simulink model "quad_control"  (R2017a)
settings: Solver=ode3  StartTime=0.0  StopTime=100  FixedStep=0.01  RelTol=1e-3  EnableMultiTasking=on
values from neighbouring files (symbols this model uses):
  g = 9.8    [init.m]
  m = 0.445    [init.m]
undefined symbols (not defined in the file or in its folder): allocate, altitude_control, attitude_control, fault_estimate, faults, model, position_control, sliding_var, sliding_var_z
libraries: simulink x2
settings Model: Creator=smishra  LastModifiedBy=Bharath
settings DataIOCC: LimitDataPoints=on  SaveFormat=Array  Refine=5
settings OptimizationCC: LifeSpan=inf
settings DebuggingCC: SFUnexpectedBacktrackingDiag=warning  SFNoUnconditionalDefaultTransitionDiag=warning  SFExecutionAtInitializationDiag=none
settings HardwareCC: ProdBitPerPointer=32  ProdBitPerSizeT=32  ProdBitPerPtrDiffT=32  ProdLargestAtomicFloat=None  ProdIntDivRoundTo=Undefined  ProdEndianess=Unspecified  ProdWordSize=32  ProdHWDeviceType=32-bit Generic
settings ModelReferenceCC: PropagateSignalLabelsOutOfModel=off
settings GRTTargetCC: TargetLangStandard=C89/C90 (ANSI)  GeneratePreprocessorConditionals=Disable all
settings ConfigComp: CovMetricSettings=dw  CovHtmlReporting=on  CovSaveCumulativeToWorkspaceVar=on  CovSaveSingleToWorkspaceVar=on  CovExternalEMLEnable=off

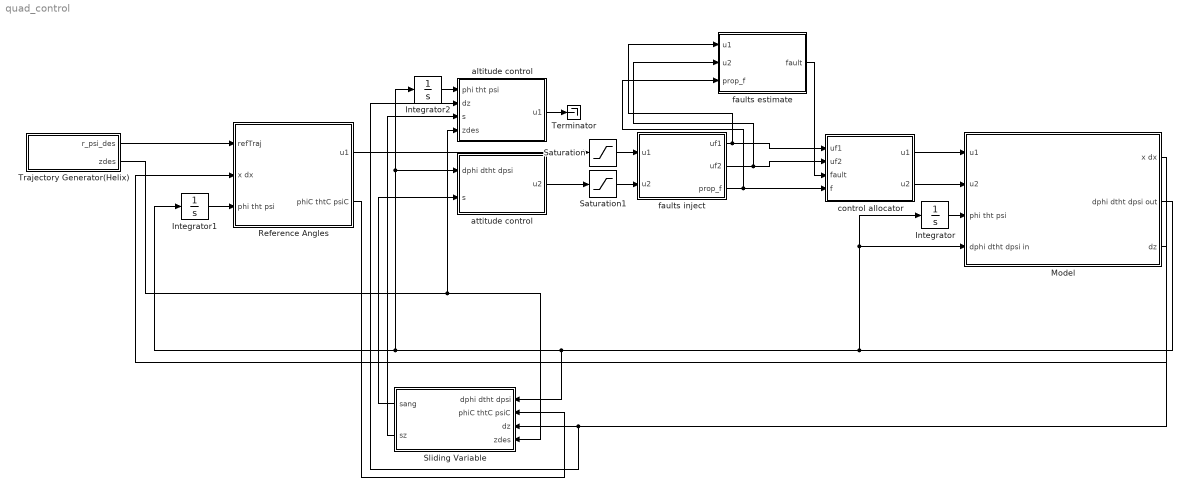
== system quad_control ==
  Integrator : Integrator
  Integrator1 : Integrator
  Integrator2 : Integrator
  Model : Subsystem
  Reference Angles : Subsystem
  Saturation : Saturate  UpperLimit=2*m*g  LowerLimit=0
  Saturation1 : Saturate  UpperLimit=0.2  LowerLimit=-0.2
  Sliding Variable : Subsystem
  Terminator : Terminator
  Trajectory Generator(Helix) : Subsystem
  altitude control : Subsystem
  attitude control : Subsystem
  control allocator : Subsystem
  faults estimate : Subsystem
  faults inject : Subsystem
  wires:
  Trajectory Generator(Helix)/1(r_psi_des) -> Reference Angles/1(refTraj)
  Model/2(dphi dtht dpsi out) -> Model/4(dphi dtht dpsi in), Integrator/1, Sliding Variable/1(dphi dtht dpsi), Integrator1/1, attitude control/1(dphi dtht dpsi), Integrator2/1
  Integrator/1 -> Model/3(phi tht psi)
  Integrator1/1 -> Reference Angles/3(phi tht psi)
  Model/1(x dx) -> Reference Angles/2(x dx)
  Sliding Variable/1(sang) -> attitude control/2(s)
  Reference Angles/2(phiC thtC psiC) -> Sliding Variable/2(phiC thtC psiC)
  Reference Angles/1(u1) -> Saturation/1
  attitude control/1(u2) -> Saturation1/1
  Trajectory Generator(Helix)/2(zdes) -> altitude control/4(zdes), Sliding Variable/4(zdes)
  Model/3(dz) -> altitude control/2(dz), Sliding Variable/3(dz)
  Sliding Variable/2(sz) -> altitude control/3(s)
  altitude control/1(u1) -> Terminator/1
  Integrator2/1 -> altitude control/1(phi tht psi)
  Saturation/1 -> faults inject/1(u1)
  Saturation1/1 -> faults inject/2(u2)
  control allocator/1(u1) -> Model/1(u1)
  control allocator/2(u2) -> Model/2(u2)
  faults estimate/1(fault) -> control allocator/3(fault)
  faults inject/1(uf1) -> faults estimate/1(u1), control allocator/1(uf1)
  faults inject/2(uf2) -> faults estimate/2(u2), control allocator/2(uf2)
  faults inject/3(prop_f) -> control allocator/4(f), faults estimate/3(prop_f)

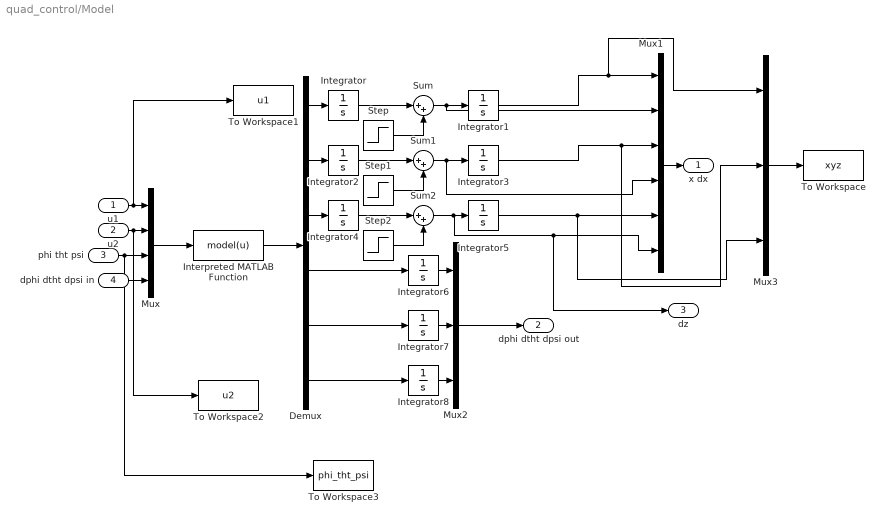
== system quad_control/Model ==
  u1 : Inport
  u2 : Inport  Port=2
  phi tht psi : Inport  Port=3
  dphi dtht dpsi in : Inport  Port=4
  Demux : Demux  Outputs=6
  Integrator{,1..2,4,6..8} (7 alike) : Integrator
  Integrator3 : Integrator  InitialCondition=8
  Integrator5 : Integrator  InitialCondition=8
  Interpreted MATLAB Function : MATLABFcn  MATLABFcn=model(u)  OutputDimensions=6
  Mux : Mux
  Mux1 : Mux  Inputs=6
  Mux2 : Mux  Inputs=3
  Mux3 : Mux  Inputs=3
  Step : Step  Time=025  After=0  SampleTime=0
  Step1 : Step  Time=25  After=0  SampleTime=0
  Step2 : Step  Time=25  After=0  SampleTime=0
  Sum : Sum  Inputs=|++
  Sum1 : Sum  Inputs=|++
  Sum2 : Sum  Inputs=|++
  To Workspace : ToWorkspace  VariableName=xyz  SampleTime=-1
  To Workspace1 : ToWorkspace  VariableName=u1  SampleTime=-1
  To Workspace2 : ToWorkspace  VariableName=u2  SampleTime=-1
  To Workspace3 : ToWorkspace  VariableName=phi_tht_psi  SampleTime=-1
  x dx : Outport
  dphi dtht dpsi out : Outport  Port=2
  dz : Outport  Port=3
  wires:
  Integrator5/1 -> Mux3/3, Mux1/5
  Mux2/1 -> dphi dtht dpsi out/1
  Mux1/1 -> x dx/1
  Mux/1 -> Interpreted MATLAB Function/1
  Integrator3/1 -> Mux3/2, Mux1/3
  Demux/3 -> Integrator4/1
  Demux/1 -> Integrator/1
  Integrator1/1 -> Mux3/1, Mux1/1
  Integrator7/1 -> Mux2/2
  Interpreted MATLAB Function/1 -> Demux/1
  Integrator8/1 -> Mux2/3
  Demux/2 -> Integrator2/1
  Integrator6/1 -> Mux2/1
  phi tht psi/1 -> Mux/3, To Workspace3/1
  Mux3/1 -> To Workspace/1
  u1/1 -> To Workspace1/1, Mux/1
  u2/1 -> To Workspace2/1, Mux/2
  dphi dtht dpsi in/1 -> Mux/4
  Demux/4 -> Integrator6/1
  Demux/5 -> Integrator7/1
  Demux/6 -> Integrator8/1
  Integrator/1 -> Sum/1
  Sum/1 -> Mux1/2, Integrator1/1
  Integrator2/1 -> Sum1/1
  Sum1/1 -> Mux1/4, Integrator3/1
  Integrator4/1 -> Sum2/1
  Sum2/1 -> dz/1, Mux1/6, Integrator5/1
  Step/1 -> Sum/2
  Step1/1 -> Sum1/2
  Step2/1 -> Sum2/2

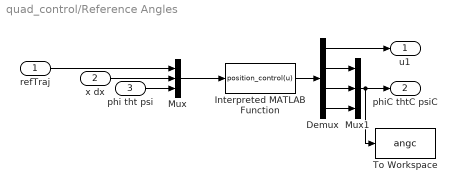
== system quad_control/Reference Angles ==
  refTraj : Inport
  x dx : Inport  Port=2
  phi tht psi : Inport  Port=3
  Demux : Demux
  Interpreted MATLAB Function : MATLABFcn  MATLABFcn=position_control(u)  OutputDimensions=4
  Mux : Mux  Inputs=3
  Mux1 : Mux  Inputs=3
  To Workspace : ToWorkspace  VariableName=angc  SampleTime=-1
  u1 : Outport
  phiC thtC psiC : Outport  Port=2
  wires:
  Mux/1 -> Interpreted MATLAB Function/1
  refTraj/1 -> Mux/1
  x dx/1 -> Mux/2
  phi tht psi/1 -> Mux/3
  Interpreted MATLAB Function/1 -> Demux/1
  Demux/1 -> u1/1
  Demux/2 -> Mux1/1
  Demux/3 -> Mux1/2
  Demux/4 -> Mux1/3
  Mux1/1 -> To Workspace/1, phiC thtC psiC/1

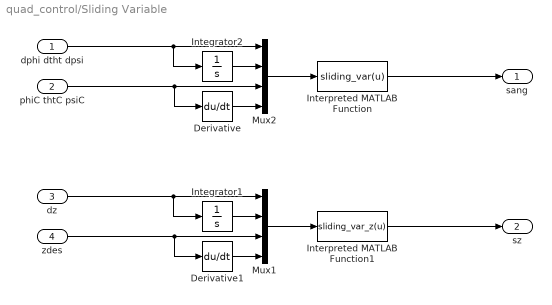
== system quad_control/Sliding Variable ==
  dphi dtht dpsi : Inport
  phiC thtC psiC : Inport  Port=2
  dz : Inport  Port=3
  zdes : Inport  Port=4
  Derivative : Derivative
  Derivative1 : Derivative
  Integrator1 : Integrator
  Integrator2 : Integrator
  Interpreted MATLAB Function : MATLABFcn  MATLABFcn=sliding_var(u)  OutputDimensions=3
  Interpreted MATLAB Function1 : MATLABFcn  MATLABFcn=sliding_var_z(u)  OutputDimensions=1
  Mux1 : Mux
  Mux2 : Mux
  sang : Outport
  sz : Outport  Port=2
  wires:
  Integrator2/1 -> Mux2/2
  Mux2/1 -> Interpreted MATLAB Function/1
  dphi dtht dpsi/1 -> Integrator2/1, Mux2/1
  Interpreted MATLAB Function/1 -> sang/1
  phiC thtC psiC/1 -> Derivative/1, Mux2/3
  Derivative/1 -> Mux2/4
  Integrator1/1 -> Mux1/2
  Mux1/1 -> Interpreted MATLAB Function1/1
  Interpreted MATLAB Function1/1 -> sz/1
  dz/1 -> Integrator1/1, Mux1/1
  zdes/1 -> Derivative1/1, Mux1/3
  Derivative1/1 -> Mux1/4

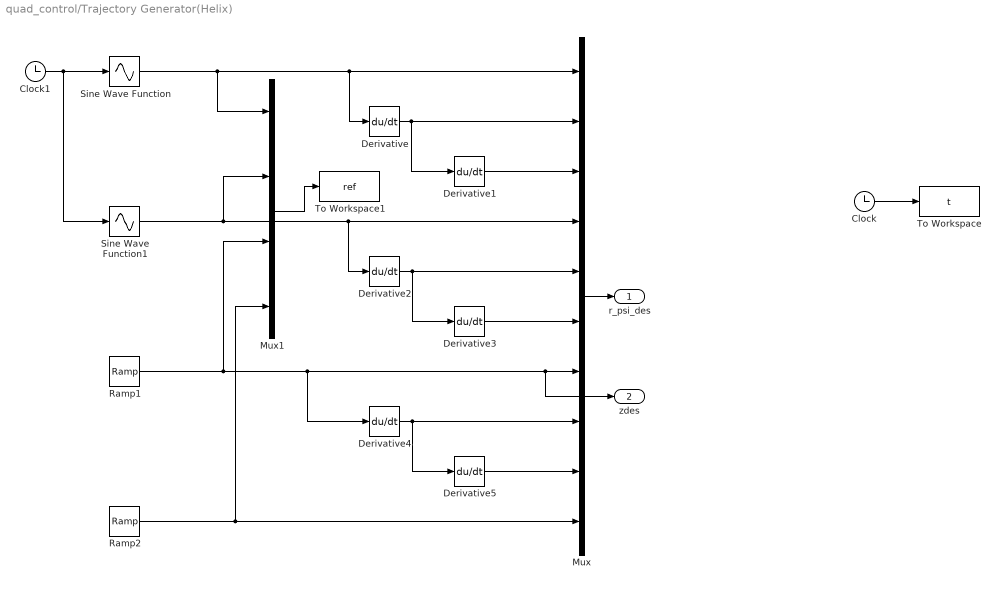
== system quad_control/Trajectory Generator(Helix) ==
  Clock : Clock
  Clock1 : Clock
  Derivative{,1..5} (6 alike) : Derivative
  Mux : Mux  Inputs=10
  Mux1 : Mux
  Ramp1 : simulink/Sources/Ramp  slope=-0.2  start=0  X0=8
  Ramp2 : simulink/Sources/Ramp  slope=0  start=0  X0=0
  Sine Wave Function : Sin  TimeSource=Use external signal  Amplitude=8  Frequency=0.1  SampleTime=0
  Sine Wave Function1 : Sin  TimeSource=Use external signal  Amplitude=8  Frequency=0.1  Phase=pi/2  SampleTime=0
  To Workspace : ToWorkspace  VariableName=t  SampleTime=-1
  To Workspace1 : ToWorkspace  VariableName=ref  SampleTime=-1
  r_psi_des : Outport
  zdes : Outport  Port=2
  wires:
  Derivative2/1 -> Mux/5, Derivative3/1
  Derivative4/1 -> Mux/8, Derivative5/1
  Derivative/1 -> Mux/2, Derivative1/1
  Derivative1/1 -> Mux/3
  Derivative3/1 -> Mux/6
  Derivative5/1 -> Mux/9
  Sine Wave Function/1 -> Mux1/1, Mux/1, Derivative/1
  Ramp2/1 -> Mux1/4, Mux/10
  Mux/1 -> r_psi_des/1
  Clock/1 -> To Workspace/1
  Clock1/1 -> Sine Wave Function1/1, Sine Wave Function/1
  Ramp1/1 -> Mux1/3, Derivative4/1, zdes/1, Mux/7
  Mux1/1 -> To Workspace1/1
  Sine Wave Function1/1 -> Mux1/2, Derivative2/1, Mux/4

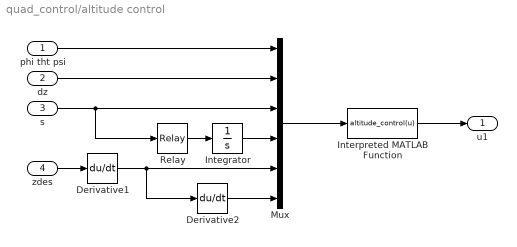
== system quad_control/altitude control ==
  phi tht psi : Inport
  dz : Inport  Port=2
  s : Inport  Port=3
  zdes : Inport  Port=4
  Derivative1 : Derivative
  Derivative2 : Derivative
  Integrator : Integrator
  Interpreted MATLAB Function : MATLABFcn  MATLABFcn=altitude_control(u)  OutputDimensions=1
  Mux : Mux  Inputs=6
  Relay : Relay
  u1 : Outport
  wires:
  Mux/1 -> Interpreted MATLAB Function/1
  Interpreted MATLAB Function/1 -> u1/1
  phi tht psi/1 -> Mux/1
  s/1 -> Mux/3, Relay/1
  Relay/1 -> Integrator/1
  Integrator/1 -> Mux/4
  dz/1 -> Mux/2
  zdes/1 -> Derivative1/1
  Derivative1/1 -> Derivative2/1, Mux/5
  Derivative2/1 -> Mux/6

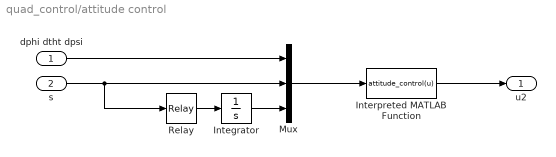
== system quad_control/attitude control ==
  dphi dtht dpsi : Inport
  s : Inport  Port=2
  Integrator : Integrator
  Interpreted MATLAB Function : MATLABFcn  MATLABFcn=attitude_control(u)  OutputDimensions=3
  Mux : Mux  Inputs=3
  Relay : Relay
  u2 : Outport
  wires:
  Mux/1 -> Interpreted MATLAB Function/1
  Interpreted MATLAB Function/1 -> u2/1
  dphi dtht dpsi/1 -> Mux/1
  s/1 -> Relay/1, Mux/2
  Relay/1 -> Integrator/1
  Integrator/1 -> Mux/3

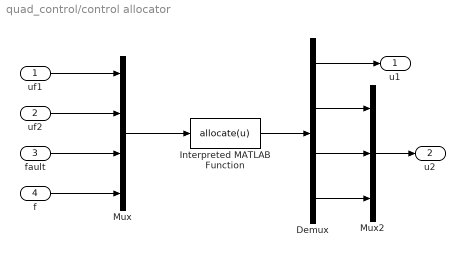
== system quad_control/control allocator ==
  uf1 : Inport
  uf2 : Inport  Port=2
  fault : Inport  Port=3
  f : Inport  Port=4
  Demux : Demux
  Interpreted MATLAB Function : MATLABFcn  MATLABFcn=allocate(u)  OutputDimensions=4
  Mux : Mux
  Mux2 : Mux  Inputs=3
  u1 : Outport
  u2 : Outport  Port=2
  wires:
  Mux/1 -> Interpreted MATLAB Function/1
  Interpreted MATLAB Function/1 -> Demux/1
  Mux2/1 -> u2/1
  uf1/1 -> Mux/1
  uf2/1 -> Mux/2
  fault/1 -> Mux/3
  f/1 -> Mux/4
  Demux/2 -> Mux2/1
  Demux/3 -> Mux2/2
  Demux/4 -> Mux2/3
  Demux/1 -> u1/1

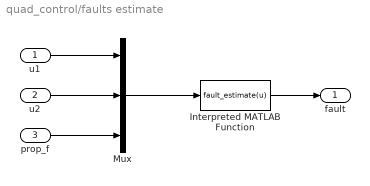
== system quad_control/faults estimate ==
  u1 : Inport
  u2 : Inport  Port=2
  prop_f : Inport  Port=3
  Interpreted MATLAB Function : MATLABFcn  MATLABFcn=fault_estimate(u)  OutputDimensions=4
  Mux : Mux  Inputs=3
  fault : Outport
  wires:
  Mux/1 -> Interpreted MATLAB Function/1
  u1/1 -> Mux/1
  u2/1 -> Mux/2
  prop_f/1 -> Mux/3
  Interpreted MATLAB Function/1 -> fault/1

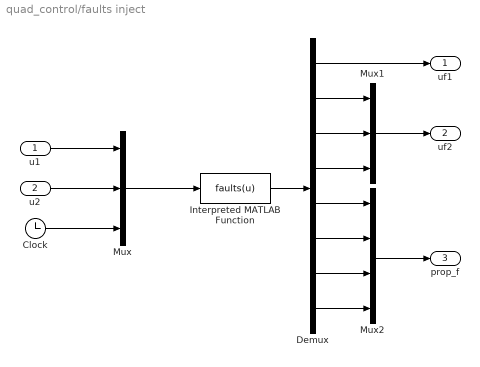
== system quad_control/faults inject ==
  u1 : Inport
  u2 : Inport  Port=2
  Clock : Clock
  Demux : Demux  Outputs=8
  Interpreted MATLAB Function : MATLABFcn  MATLABFcn=faults(u)  OutputDimensions=8
  Mux : Mux  Inputs=3
  Mux1 : Mux  Inputs=3
  Mux2 : Mux
  uf1 : Outport
  uf2 : Outport  Port=2
  prop_f : Outport  Port=3
  wires:
  Mux/1 -> Interpreted MATLAB Function/1
  Interpreted MATLAB Function/1 -> Demux/1
  Demux/4 -> Mux1/3
  Demux/3 -> Mux1/2
  Demux/2 -> Mux1/1
  Demux/8 -> Mux2/4
  Demux/7 -> Mux2/3
  Demux/6 -> Mux2/2
  Demux/5 -> Mux2/1
  Demux/1 -> uf1/1
  Mux2/1 -> prop_f/1
  Mux1/1 -> uf2/1
  u1/1 -> Mux/1
  u2/1 -> Mux/2
  Clock/1 -> Mux/3
